simulink model "p1"  (R2019b)
settings: Solver=VariableStepAuto  StartTime=0.0  StopTime=100  RelTol=1e-3
values from neighbouring files (symbols this model uses):
  A = [ 0             0         1              0 ... (first row only)    [control_p1.m]
  B = [0; 0; 1; 0]    [control_p1.m]
  C = [1 0 0 0]    [control_p1.m]
  X = [0.5; 1; -0.1; 0.5]    [control_p1.m]
settings Model: Creator=samel  LastModifiedBy=sharathchandra
settings DataIOCC: ReturnWorkspaceOutputs=off
settings DebuggingCC: ArithmeticOperatorsInVariantConditions=warning
settings SFSimCC: CustomCodeUndefinedFunction=UseInterfaceOnly

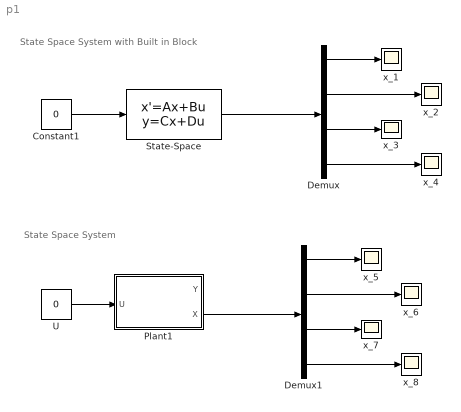
== system p1 ==
  note: State Space System
  note: State Space System with Built in Block
  Constant1 : Constant  Value=0
  Demux : Demux
  Demux1 : Demux
  Plant1 : Subsystem
  State-Space : StateSpace  A=A  B=B  C=eye(4)  D=[0; 0; 0;0]  InitialCondition=X  ContinuousStateAttributes={'x_1','x_2','x_3','x_4'}
  U : Constant  Value=0
  x_{1..8} (8 alike) : Scope
  wires:
  Demux/3 -> x_3/1
  Demux/2 -> x_2/1
  Demux/4 -> x_4/1
  Demux/1 -> x_1/1
  State-Space/1 -> Demux/1
  Demux1/3 -> x_7/1
  Demux1/4 -> x_8/1
  Demux1/2 -> x_6/1
  Demux1/1 -> x_5/1
  Plant1/2(X) -> Demux1/1
  Constant1/1 -> State-Space/1
  U/1 -> Plant1/1(U)

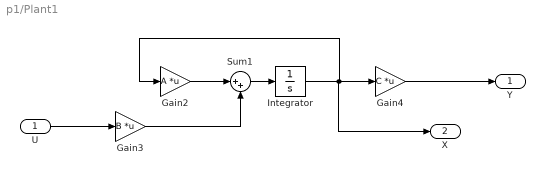
== system p1/Plant1 ==
  U : Inport
  Gain2 : Gain  Gain=A  Multiplication=Matrix(K*u)
  Gain3 : Gain  Gain=B  Multiplication=Matrix(K*u)
  Gain4 : Gain  Gain=C  Multiplication=Matrix(K*u)
  Integrator : Integrator  InitialCondition=X
  Sum1 : Sum  Inputs=|++
  Y : Outport  VectorParamsAs1DForOutWhenUnconnected=off
  X : Outport  Port=2  VectorParamsAs1DForOutWhenUnconnected=off
  wires:
  Gain2/1 -> Sum1/1
  Gain4/1 -> Y/1
  Integrator/1 -> X/1, Gain2/1, Gain4/1
  Sum1/1 -> Integrator/1
  Gain3/1 -> Sum1/2
  U/1 -> Gain3/1
